simulink model "mod_2R2010a"  (Simulink 7.5)
settings: Solver=ode45  StartTime=0.0  StopTime=10.0  RelTol=1e-3
settings Model: Creator=Professor Dingyu Xue  LastModifiedBy=Professor Dingyu Xue
settings OptimizationCC: InlineParams=on

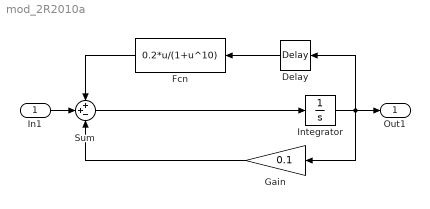
== system mod_2R2010a ==
  In1 : Inport
  Delay : TransportDelay  BufferSize=10240
  Fcn : Fcn  Expr=0.2*u/(1+u^10)
  Gain : Gain  Gain=0.1
  Integrator : Integrator
  Sum : Sum  Inputs=++-
  Out1 : Outport
  wires:
  Integrator/1 -> Out1/1, Delay/1, Gain/1
  Sum/1 -> Integrator/1
  Gain/1 -> Sum/3
  In1/1 -> Sum/2
  Delay/1 -> Fcn/1
  Fcn/1 -> Sum/1
